simulink model "mOneLossMap3D"  (R2021b)
settings: Solver=VariableStepAuto  StartTime=0.0  StopTime=10.0  RelTol=1e-3
values from neighbouring files (symbols this model uses):
  speedVal = SpeedMat(end,end)    [tLossMaps.m]    (also in tLossMapsWithDCV.m = SpeedVec(end))
  torqueVal = ShaftTorqueMat(end,end)    [tLossMaps.m]    (also in tLossMapsWithDCV.m = TorqueVec(end))
  xVec = linspace(xMin, xMax, xLen)    [tLossMaps.m]    (also in tLossMapsWithDCV.m = linspace(min(xMat(:)), max(xMat(:)), nx))
  yVec = linspace(yMin, yMax, yLen)    [tLossMaps.m]    (also in tLossMapsWithDCV.m = linspace(min(yMat(:)), max(yMat(:)), ny))
  zgMat = zInterpolant(xgrid, ygrid)    [tLossMaps.m]
  zVec = linspace(min(zMat(:)), max(zMat(:)), nz)    [tLossMapsWithDCV.m]
undefined symbols (not defined in the file or in its folder): voltageVal
settings Model: Creator=agonzale  LastModifiedBy=agonzale

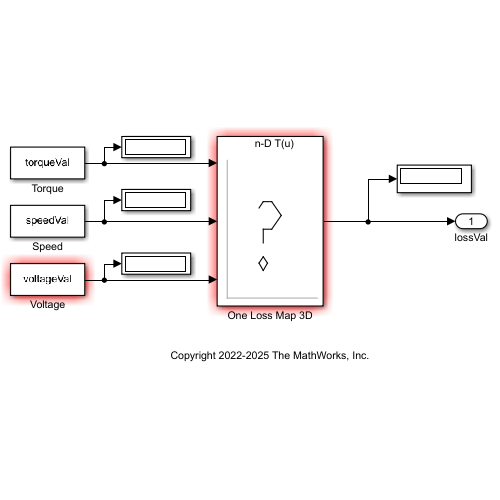
[thumbnail: Simulink's stored preview of the top-level diagram]
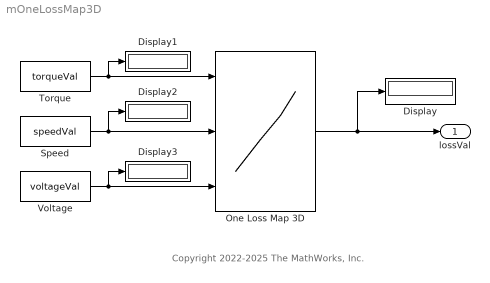
== system mOneLossMap3D ==
  note: Copyright 2022-2025 The MathWorks, Inc.
  Display{,1..3} (4 alike) : Display
  One Loss Map 3D : Lookup_n-D  NumberOfTableDimensions=3  BreakpointsForDimension1=xVec  BreakpointsForDimension2=yVec  BreakpointsForDimension3=zVec  Table=zgMat  ExtrapMethod=Clip  UseLastTableValue=on  InternalRulePriority=Speed  RndMeth=Simplest  InputSameDT=on
      settings: InputPortMap=u0,u1,u2
  Speed : Constant  Value=speedVal
  Torque : Constant  Value=torqueVal
  Voltage : Constant  Value=voltageVal
  lossVal : Outport
  wires:
  Torque/1 -> One Loss Map 3D/1, Display1/1
  Speed/1 -> One Loss Map 3D/2, Display2/1
  One Loss Map 3D/1 -> Display/1, lossVal/1
  Voltage/1 -> Display3/1, One Loss Map 3D/3
